simulink subsystem "Orbit_sim_measurement"  (R2024a)
settings: Solver=VariableStepAuto  StartTime=0.0  StopTime=10.0  RelTol=1e-3
undefined symbols (not defined in the file or in its folder): J1, J2, J3
settings Model: Creator=ruimi  LastModifiedBy=alenachan

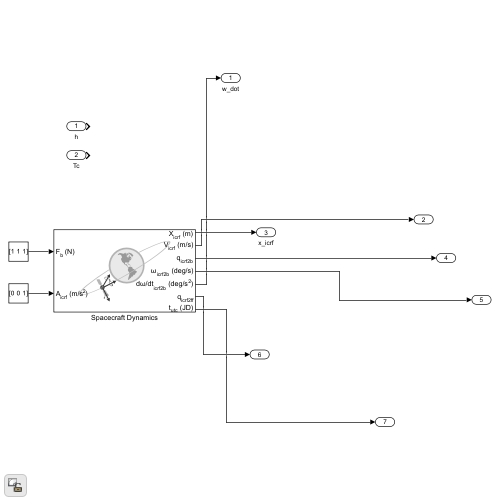
[thumbnail: Simulink's stored preview of the top-level diagram]
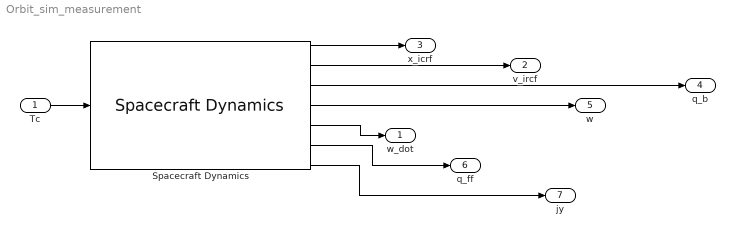
== system Orbit_sim_measurement ==
  Tc : Inport
  Spacecraft Dynamics : SpacecraftDynamics  forcesIn=off  startDate=2458850.00000058  mass=m  inertia=[J1,0,0;0,J2,0;0,0,J3]  stateFormatNum=ICRF state vector  semiMajorAxis=8413000  eccentricity=0.025  inclination=Orbit_Incl  raan=299.4750  argPeriapsis=347.2333  trueAnomaly=109  inertialPosition=[3649562.45420845 3308533.31475011 -4676471.32255767]  inertialVelocity=[-2751.03166056909 6666.19000105801 2573.69769194449]  attitudeFrame=NED  attitude=[-0.837416846202256;0.0356568317608846;-0.355955388615428;0.413227996826307]  attitudeRate=[-148025.956674316;-259656.699449149;192869.781839077]  outputAngAccel=on  earthSH=EGM96  outputTransform=on  useDrag=on  useSRP=on
  w_dot : Outport
  v_ircf : Outport  Port=2
  x_icrf : Outport  Port=3
  q_b : Outport  Port=4
  w : Outport  Port=5
  q_ff : Outport  Port=6
  jy : Outport  Port=7
  wires:
  Spacecraft Dynamics/5 -> w_dot/1
  Spacecraft Dynamics/4 -> w/1
  Spacecraft Dynamics/7 -> jy/1
  Spacecraft Dynamics/2 -> v_ircf/1
  Spacecraft Dynamics/1 -> x_icrf/1
  Spacecraft Dynamics/6 -> q_ff/1
  Spacecraft Dynamics/3 -> q_b/1
  Tc/1 -> Spacecraft Dynamics/1
